simulink model "wind_turb_asyn"  (R2021b)
settings: Solver=VariableStepAuto  StartTime=0.0  StopTime=10.0  RelTol=1e-3
InitFcn:
  | sampling=0.1;
undefined symbols (not defined in the file): sigbuilder_block
settings Model: Creator=Omar  LastModifiedBy=Omar

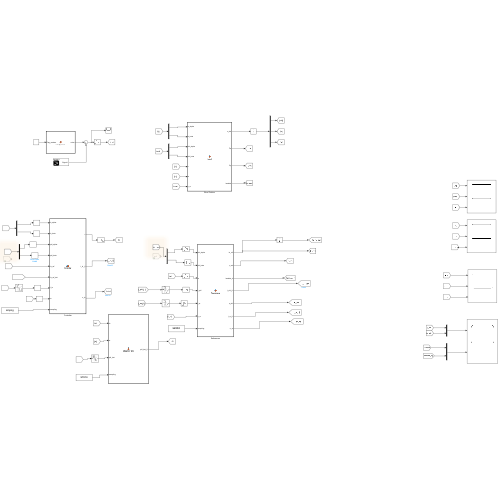
[thumbnail: Simulink's stored preview of the top-level diagram]
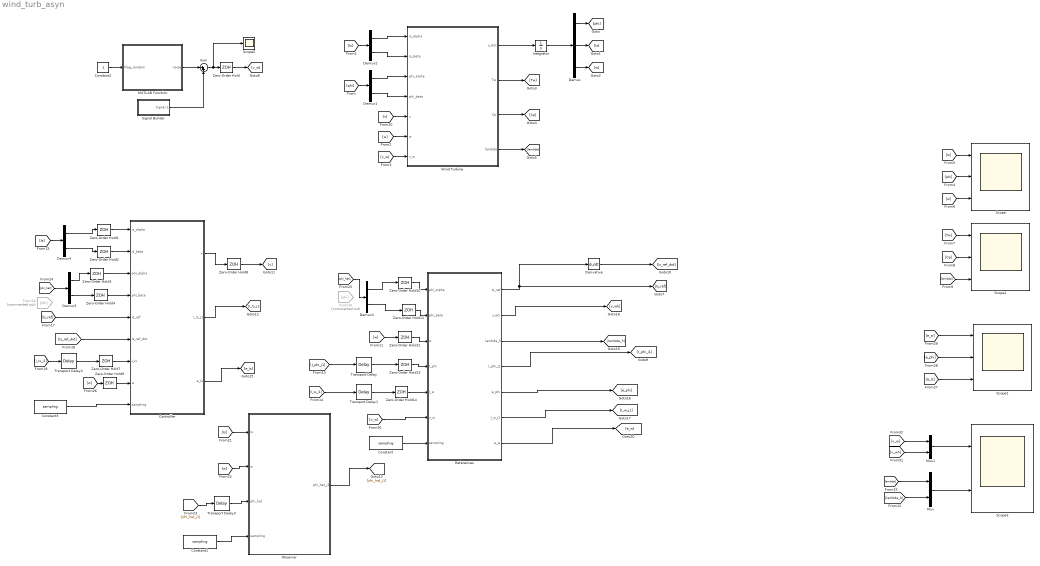
== system wind_turb_asyn ==
  Constant : Constant  Value=sampling
  Constant1 : Constant  Value=sampling
  Constant2 : Constant
  Constant3 : Constant  Value=sampling
  Controller : MATLAB Function  TreatAsAtomicUnit=on
  Demux : Demux  Outputs=3
  Demux{1..5} (5 alike) : Demux  Outputs=2
  Derivative : Derivative
  From10 : From  Commented=on  GotoTag=phi
  From16 : From  Commented=on  GotoTag=phi
  Integrator : Integrator  InitialCondition=[0.5;0.5;2000;2000;1.5]
  MATLAB Function : MATLAB Function  TreatAsAtomicUnit=on
  Mux : Mux  Inputs=2
  Mux1 : Mux  Inputs=2
  Observer : MATLAB Function  TreatAsAtomicUnit=on
  References : MATLAB Function  TreatAsAtomicUnit=on
  Scope : Scope  NumInputPorts=3
  Scope1 : Scope  NumInputPorts=3
  Scope2 : Scope  NumInputPorts=3
  Scope3 : Scope  NumInputPorts=2
  Scope5 : Scope
  Signal Builder : Subsystem  Tag=STV Subsys  LoadFcn=sigbuilder_block('load');  StartFcn=sigbuilder_block('start');  StopFcn=sigbuilder_block('stop');  ClipboardFcn=sigbuilder_block('clipboard');  mask(Sigbuilder block){tuvar=[0:10]}
      mask help: Simulink:masks:SigbuilderBlock_MD
      mask init:
      | if ~strcmp(get_param(bdroot(gcbh),'SimulationStatus'),'stopped') tuvar = sigbuilder_block('maskInit'); end
      settings: CopyFcn=sigbuilder_block('copy');  DeleteFcn=sigbuilder_block('delete');  ModelCloseFcn=sigbuilder_block('modelClose');  PreSaveFcn=sigbuilder_block('preSave');  PauseFcn=sigbuilder_block('pause');  ContinueFcn=sigbuilder_block('continue');  NameChangeFcn=sigbuilder_block('namechange');  OpenFcn=sigbuilder_block('open',[5.4 33 1141.2 514.8 ]);  CloseFcn=sigbuilder_block('close');
      mask Display: plot(0, 0, 100, 100,[2, 2, 32, 32, 2], [68, 8, 8, 68, 68],[32, 2], [38, 38], [32, 19, 2],[53, 60, 44], [32, 17, 17, 2],[16, 16, 31, 31]);txt = getActiveGroup(gcbh);text(2, 100, txt,'verticalAlignment', 'top');
  Sum : Sum  Inputs=|++
  Transport Delay : TransportDelay  DelayTime=sampling
  Transport Delay1 : TransportDelay  DelayTime=sampling
  Transport Delay2 : TransportDelay  DelayTime=sampling  InitialOutput=[0;0]
  Transport Delay3 : TransportDelay  DelayTime=sampling  InitialOutput=[0.25;0.25]
  Wind Turbine : MATLAB Function  TreatAsAtomicUnit=on
  Zero-Order Hold{,1..4,7..14} (13 alike) : ZeroOrderHold  SampleTime=sampling
  wires:
  Wind Turbine/1(x_dot) -> Integrator/1
  Integrator/1 -> Demux/1
  Demux/1 -> [phi]
  Demux/2 -> [Is]
  Demux/3 -> [w]
  [w] -> Wind Turbine/6(w)
  Demux1/2 -> Wind Turbine/4(phi_beta)
  Demux2/2 -> Wind Turbine/2(is_beta)
  Demux2/1 -> Wind Turbine/1(is_alpha)
  Wind Turbine/2(Tw) -> [Tw]
  Wind Turbine/3(Cp) -> [Cp]
  Wind Turbine/4(lambda) -> [lambda]
  [Is] -> Demux2/1
  Demux1/1 -> Wind Turbine/3(phi_alpha)
  [phi] -> Demux1/1
  Sum/1 -> Scope5/1, Zero-Order Hold/1
  MATLAB Function/1(noise) -> Sum/1
  Zero-Order Hold/1 -> [v_w]
  Constant2/1 -> MATLAB Function/1(Flag_random)
  Signal Builder/1(Signal 1) -> Sum/2
  [v_w] -> Wind Turbine/7(v_w)
  [v] -> Wind Turbine/5(v)
  [phi] -> Scope/2
  [Is] -> Scope/1
  [w] -> Scope/3
  Demux3/1 -> Zero-Order Hold10/1
  Demux3/2 -> Zero-Order Hold11/1
  [w] -> Zero-Order Hold12/1
  References/1(Is_ref) -> Derivative/1, [Is_ref]
  [Is] -> Demux4/1
  Demux4/1 -> Zero-Order Hold1/1
  Demux4/2 -> Zero-Order Hold2/1
  Demux5/1 -> Zero-Order Hold3/1
  Controller/2(I_Is_j1) -> [I_Is_j1]
  [w] -> Observer/2(w)
  [Is] -> Observer/1(Is)
  [phi_hat] -> Demux3/1
  [phi_hat] -> Demux5/1
  [e_w] -> Scope2/1
  [e_phi] -> Scope2/2
  [e_Is] -> Scope2/3
  [v_w] -> References/6(v_w)
  References/4(I_phi_j1) -> [I_phi_j1]
  References/3(lambda_h) -> [lambda_h]
  References/2(v_wh) -> [v_wh]
  [lambda_h] -> Mux/2
  [lambda] -> Mux/1
  [v_wh] -> Mux1/2
  [v_w] -> Mux1/1
  Mux1/1 -> Scope3/1
  Mux/1 -> Scope3/2
  Zero-Order Hold1/1 -> Controller/1(is_alpha)
  Zero-Order Hold2/1 -> Controller/2(is_beta)
  Zero-Order Hold3/1 -> Controller/3(phi_alpha)
  Demux5/2 -> Zero-Order Hold4/1
  Zero-Order Hold4/1 -> Controller/4(phi_beta)
  [Is_ref] -> Controller/5(Is_ref)
  Zero-Order Hold7/1 -> Controller/7(I_Is)
  [w] -> Zero-Order Hold9/1
  Zero-Order Hold9/1 -> Controller/8(w)
  Controller/1(v) -> Zero-Order Hold8/1
  Zero-Order Hold8/1 -> [v]
  Zero-Order Hold10/1 -> References/1(phi_alpha)
  Zero-Order Hold11/1 -> References/2(phi_beta)
  Zero-Order Hold12/1 -> References/3(w)
  Zero-Order Hold13/1 -> References/4(I_phi)
  Zero-Order Hold14/1 -> References/5(I_w)
  Derivative/1 -> [Is_ref_dot]
  [I_phi_j1] -> Transport Delay/1
  Transport Delay/1 -> Zero-Order Hold13/1
  References/5(e_phi) -> [e_phi]
  References/6(I_w_j1) -> [I_w_j1]
  References/7(e_w) -> [e_w]
  [I_w_j1] -> Transport Delay1/1
  Transport Delay1/1 -> Zero-Order Hold14/1
  Controller/3(e_Is) -> [e_Is]
  [I_Is_j1] -> Transport Delay2/1
  Transport Delay2/1 -> Zero-Order Hold7/1
  [phi_hat_j1] -> Transport Delay3/1
  Transport Delay3/1 -> Observer/3(phi_hat)
  Observer/1(phi_hat_j1) -> [phi_hat_j1]
  Constant/1 -> References/7(sampling)
  Constant1/1 -> Observer/4(sampling)
  Constant3/1 -> Controller/9(sampling)
  [Is_ref_dot] -> Controller/6(Is_ref_dot)
  [Tw] -> Scope1/1
  [Cp] -> Scope1/2
  [lambda] -> Scope1/3

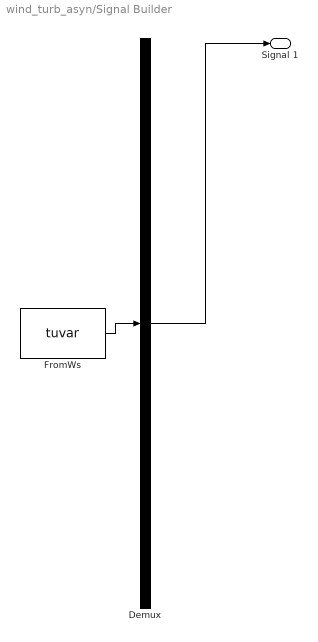
== system wind_turb_asyn/Signal Builder ==
  Demux : Demux  Tag=STV Demux  Outputs=1
      settings: DisplayOption=none
  FromWs : FromWorkspace  Tag=STV FromWs  VariableName=tuvar
      SigBuilderData=|
      | common.afterFinalStr = 'Extrapolate'
      | common.sampleTime = 0
      | dataSet.timeRange = [0 10]
      | dataSet.name = 'Group 1'
      | sbobj.Groups.Name = 'Group 1'
      | sbobj.Groups.Signals.Name = 'Signal 1'
      | sbobj.Groups.Signals.XData = [0 1.9 2.9 8 8.2 10]
      | sbobj.Groups.Signals.YData = [7 7 9.4 9.4 9 9]
  Signal 1 : Outport  Tag=STV Outport
  wires:
  Demux/1 -> Signal 1/1
  FromWs/1 -> Demux/1

== matlab function wind_turb_asyn/MATLAB Function ==
  data: Flag_random input; noise output
function noise  = wind_noise(Flag_random)
noise=Flag_random*0.005*randi([-10,10]);
end

== matlab function wind_turb_asyn/Wind Turbine ==
  data: is_alpha input; x_dot output; is_beta input; phi_alpha input; phi_beta input; v input; w input; v_w input; Tw output; Cp output; lambda output
function [x_dot,Tw,Cp,lambda]  = model(is_alpha,is_beta,phi_alpha,phi_beta,v,w,v_w)
R=46.6;%radius of the turbine
L=1.5731e-3;
p=26;
J=34.6e3;
f=1.5e-3;
alpha=0.5;
beta=1;
gamma=1;
Lm=10;
mu=0.1;
J1=[0 -1;1 0];
Is=[is_alpha;is_beta];
phi=[phi_alpha;phi_beta];

c1=0.5176;
c2=116;
c3=0.035;
c4=5;
c5=21;
c6=0.0068;
c7=0.035;

rho=1.225;

Cp_max=0.48;

lambda=(w*R)/v_w;
C_p=c1*(c2*(1/lambda-c3)-c4)*exp(-c5*(1/lambda-c3))+c6*lambda;
if C_p>0
    Cp=C_p;
else
    Cp=0;
end

T_w=(rho*pi*R^5*Cp*w^2)/(2*lambda^3); %T_w=kw*w^2
if T_w>0
    Tw=T_w;
else
    Tw=0;
end



phi_dot=-alpha*phi+p*w*J1*phi+alpha*Lm*Is;
Is_dot=alpha*beta*phi-p*beta*w*J1*phi-gamma*Is+(v/L);
w_dot=-mu*Is'*J1*phi-(f/J)*w+(Tw/J);
x_dot=[phi_dot;Is_dot;w_dot];
end

== matlab function wind_turb_asyn/References ==
  data: phi_alpha input; phi_beta input; w input; I_phi input; Is_ref output; I_w input; v_wh output; lambda_h output; I_phi_j1 output; v_w input; e_phi output; I_w_j1 output; e_w output; sampling input
function [Is_ref,v_wh,lambda_h,I_phi_j1,e_phi,I_w_j1,e_w]  = References(phi_alpha,phi_beta,w,I_phi,I_w,v_w,sampling)
R=46.6;%radius of the turbine
L=1.5731e-3;
p=26;
J=34.6e3;
f=1.5e-3;
alpha=0.5;
beta=1;
gamma=1;
Lm=10;
mu=0.1;
J1=[0 -1;1 0];

phi=[phi_alpha;phi_beta];

c1=0.5176;
c2=116;
c3=0.035;
c4=5;
c5=21;
c6=0.0068;
c7=0.035;

rho=1.225;

lambda_max=8.1;
Cp_max=0.48;

lambda=(w*R)/v_w;
C_p=c1*(c2*(1/lambda-c3)-c4)*exp(-c5*(1/lambda-c3))+c6*lambda;
if C_p>0
    Cp=C_p;
else
    Cp=0;
end

T_w=(rho*pi*R^5*Cp*w^2)/(2*lambda^3); %T_w=kw*w^2
if T_w>0
    Tw=T_w;
else
    Tw=0;
end

%% Estimation of lambda
v_wh0=7.5; % Initial value of the estimated wind velocity
lambda_h=(w*R)/v_wh0; % Initial value of the estimated tip speed ratio
C_ph=c1*(c2*(1/lambda_h-c3)-c4)*exp(-c5*(1/lambda_h-c3))+c6*lambda_h;
if C_ph>0
    Cph=C_ph;
else
    Cph=0;
end

kw0=(rho*pi*R^5*Cph)/(2*lambda_h^3);
T_w0=kw0*w^2;
if T_w0>0
    Tw0=T_w0;
else
    Tw0=0;
end
a1=c1*(-c2*c3/lambda_h-c2*(-c3*lambda_h+1)/lambda_h^2)*exp(-c5*(-c3*lambda_h+1)/lambda_h+c4)+c1*(c2*(-c3*lambda_h+1)/lambda_h-c4)*(c5*c3/lambda_h+c5*(-c3*lambda_h+1)/lambda_h^2)*exp(-c5*(-c3*lambda_h+1)/lambda_h+c4)+c6;
a2=3*(c1*(c2*(-c3*lambda_h+1)/lambda_h-c4)*exp(-c5*(-c3*lambda_h+1)/lambda_h+c4)+c6*lambda_h);
DCp=a1/lambda_h^3-a2/lambda_h^4;

kw=(rho*pi*R^5*Cp)/(2*lambda^3);
%Power measured
Pm=kw*w^3;


f_lambda=Pm-kw0*w^3;
df_lambda=-(rho*pi*R^5*w^3*DCp)/2;

N=109;
% Newton-Raphson method
for i=1:N
    lambda_h=lambda_h-f_lambda/df_lambda;
end

C_ph=c1*(c2*(1/lambda_h-c3)-c4)*exp(-c5*(1/lambda_h-c3))+c6*lambda_h;
if C_ph>0
    Cph=C_ph;
else
    Cph=0;
end
kw0=(rho*pi*R^5*Cph)/(2*lambda_h^3);
T_w0=kw0*w^2;
if T_w0>0
    Tw0=T_w0;
else
    Tw0=0;
end

v_wh=w*R/lambda_h;


%% definition of controller and references

phi_ref=1;% la norma di phi è errore è basato sulla norma di phi - questa phiref
phi_ref_dot=0;

e_phi=norm(phi)-phi_ref;
%Heuler approximation method
%I_phi_dot=e_phi;


I_phi_j1=I_phi+sampling*(e_phi);

kp_phi=10000;
ki_phi=5000;

w_ref=lambda_max*v_wh/R;

e_w=w-w_ref;

%Heuler approximation method



I_w_j1=I_w+sampling*(e_phi);
%I_w_dot=e_w;

kp_w=10000;
ki_w=5000;

w_control=[(1/(alpha*Lm))*(alpha*norm(phi)+phi_ref_dot-kp_phi*e_phi-ki_phi*I_phi)*norm(phi);
    (1/mu)*(-(f/J)*w+(T_w0/J)+(kp_w*e_w+ki_w*I_w))];
Is_ref=[phi';-phi'*J1]'*w_control;
end

== matlab function wind_turb_asyn/Controller ==
  data: is_alpha input; is_beta input; phi_alpha input; phi_beta input; Is_ref input; v output; Is_ref_dot input; I_Is input; w input; I_Is_j1 output; e_Is output; sampling input
function [v,I_Is_j1,e_Is]    = Controller(is_alpha,is_beta,phi_alpha,phi_beta,Is_ref,Is_ref_dot,I_Is,w,sampling)
R=46.6;%radius of the turbine
L=1.5731e-3;
p=26;
J=34.6e3;
f=1.5e-3;
alpha=0.5;
beta=1;
gamma=1;
Lm=10;
mu=0.1;
J1=[0 -1;1 0];
Is=[is_alpha;is_beta];
phi=[phi_alpha;phi_beta];

c1=0.5176;
c2=116;
c3=0.035;
c4=5;
c5=21;
c6=0.0068;
c7=0.035;

rho=1.225;

lambda_max=8.1;
Cp_max=0.48;
Is=[is_alpha;is_beta];

e_Is=Is-Is_ref;
%Heuler approximation method



I_Is_j1=I_Is+sampling*(e_Is);
%I_Is_dot=e_Is;

kp_Is=10000;
ki_Is=1000;

v=L*(-alpha*beta*phi+p*beta*w*J1*phi+gamma*Is+Is_ref_dot-kp_Is*e_Is-ki_Is*I_Is);


end

== matlab function wind_turb_asyn/Observer ==
  data: Is input; w input; phi_hat input; phi_hat_j1 output; sampling input
function phi_hat_j1 = Observer_phi(Is, w, phi_hat,sampling)

R=46.6;%radius of the turbine
L=1.5731e-3;
p=26;
J=34.6e3;
f=1.5e-3;
alpha=0.5;
beta=1;
gamma=1;
Lm=10;
mu=0.1;
J1=[0 -1;1 0];


c1=0.5176;
c2=116;
c3=0.035;
c4=5;
c5=21;
c6=0.0068;
c7=0.035;

rho=1.225;

lambda_max=8.1;
Cp_max=0.48;

%Euler approximation
phi_hat_j1=phi_hat+sampling*(-alpha*phi_hat+p*w*J1*phi_hat+alpha*Lm*Is);
